simulink model "P5OAAA"  (R2018a)
settings: Solver=VariableStepAuto  StartTime=0.0  StopTime=20  RelTol=1e-3
settings Model: Creator=sasm  LastModifiedBy=Oscar

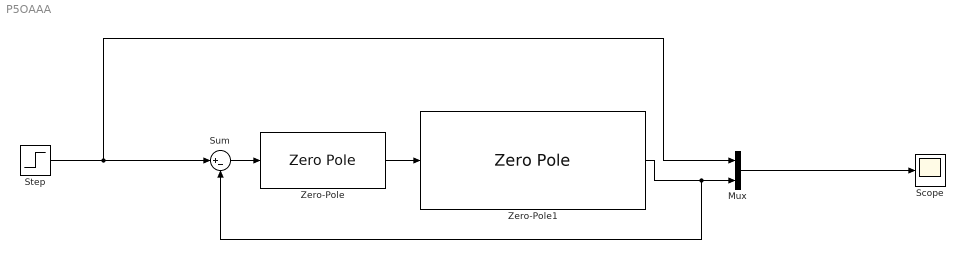
== system P5OAAA ==
  Mux : Mux  Inputs=2
  Scope : Scope
  Step : Step  SampleTime=0
  Sum : Sum  Inputs=|+-
  Zero-Pole : ZeroPole  Zeros=[-0.916]  Poles=[-3.537]  Gain=2.0002
  Zero-Pole1 : ZeroPole  Zeros=[100 -2729]  Poles=[0 -9.967 -1]  Gain=-3.6519e-05
  wires:
  Step/1 -> Sum/1, Mux/1
  Sum/1 -> Zero-Pole/1
  Mux/1 -> Scope/1
  Zero-Pole/1 -> Zero-Pole1/1
  Zero-Pole1/1 -> Sum/2, Mux/2
